simulink model "BldcClosedLoop2"  (R2020b)
settings: Solver=ode45  StartTime=0.0  StopTime=1  FixedStep=.001  RelTol=1e-3  AbsTol=1e-3  EnableMultiTasking=on
values from neighbouring files (symbols this model uses):
  c1 = 3*wmax/(t1*t1)    (= 120000)    [data_bldc_ClosedLoop2.m]
  c2 = -2*wmax/(t1*t1*t1)    (= -800000)    [data_bldc_ClosedLoop2.m]
  D = 2e-3    (= 0.002)    [data_bldc_ClosedLoop2.m]
  d1 = 3*wmax/((t3-t2)*(t3-t2))    (= 120000)    [data_bldc_ClosedLoop2.m]
  d2 = -2*wmax/((t3-t2)*(t3-t2)*(t3-t2))    (= -800000)    [data_bldc_ClosedLoop2.m]
  ep = 0.5128    [data_bldc_ClosedLoop2.m]
  Gamma_Inv = Gamma^-1    [data_bldc_ClosedLoop2.m]
  J = 2.0e-4    (= 0.0002)    [data_bldc_ClosedLoop2.m]
  k0 = p0*p1*p2    (= 1000000)    [data_bldc_ClosedLoop2.m]
  k1 = p0*p1 + p0*p2 + p1*p2    (= 30000)    [data_bldc_ClosedLoop2.m]
  k2 = p0+p1+p2    (= 300)    [data_bldc_ClosedLoop2.m]
  KI = 0*1e6    (= 0)    [data_bldc_ClosedLoop2.m]
  Kp = 1000    [data_bldc_ClosedLoop2.m]
  Rs = 0.7    [data_bldc_ClosedLoop2.m]
  t3 = t2 + t1    (= 0.7)    [data_bldc_ClosedLoop2.m]
  tau_L = 0    [data_bldc_ClosedLoop2.m]
  tdd = .1    (= 0.1)    [data_bldc_ClosedLoop2.m]
libraries: simulink x2
(part 1 of 2)
settings Model: Creator=johnchiasson  LastModifiedBy=johnchiasson
settings SolverCC: AutoScaleAbsTol=off
settings DataIOCC: LimitDataPoints=on  SaveFormat=Array  SignalLoggingSaveFormat=ModelDataLogs  ReturnWorkspaceOutputs=off  SignalLoggingName=sigsOut
settings OptimizationCC: BlockReduction=off  BooleanDataType=off  LifeSpan=inf
settings DebuggingCC: SaveWithParameterizedLinksMsg=none  UnderspecifiedInitializationDetection=Classic  MergeDetectMultiDrivingBlocksExec=none  SignalResolutionControl=TryResolveAllWithWarning  MultiTaskDSMMsg=warning  MultiTaskCondExecSysMsg=none  SFUnexpectedBacktrackingDiag=warning  SFNoUnconditionalDefaultTransitionDiag=warning  SFExecutionAtInitializationDiag=none  ArithmeticOperatorsInVariantConditions=warning
settings HardwareCC: ProdBitPerPointer=32  ProdBitPerSizeT=32  ProdBitPerPtrDiffT=32  ProdLargestAtomicFloat=None  ProdIntDivRoundTo=Undefined  ProdEndianess=Unspecified  ProdWordSize=32  ProdHWDeviceType=32-bit Generic  TargetUnknown=on
settings ModelReferenceCC: PropagateSignalLabelsOutOfModel=off
settings SFSimCC: SimUseLocalCustomCode=off  CustomCodeUndefinedFunction=UseInterfaceOnly
settings RTWCC: RTWUseLocalCustomCode=off
settings CodeAppCC: StateflowObjectComments=on
settings GRTTargetCC: TargetLangStandard=C89/C90 (ANSI)  CombineOutputUpdateFcns=off  GRTInterface=on
settings ConfigComp: CovMetricSettings=dw  CovSaveCumulativeToWorkspaceVar=on  CovSaveSingleToWorkspaceVar=on  CovExternalEMLEnable=off  CovSFcnEnable=off

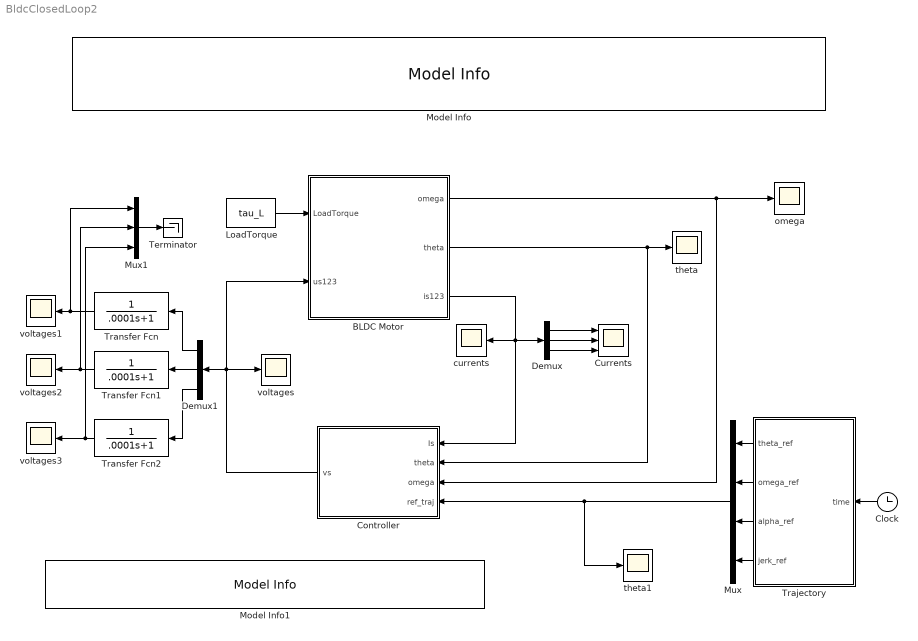
== system BldcClosedLoop2 ==
  BLDC Motor : Subsystem
  Clock : Clock
  Controller : Subsystem
  Currents : Scope  NumInputPorts=3
  Demux : Demux  Outputs=3
      settings: DisplayOption=none
  Demux1 : Demux  Outputs=3
      settings: DisplayOption=none
  LoadTorque : Constant  Value=tau_L
  Model Info : simulink/Model-Wide Utilities/Model Info  Frame=on  DisplayStringWithTags="Simulation of a Three-Phase  Trapezoidal Back EMF BLDC"  HorizontalTextAlignment=Center  LeftAlignmentValue=0.5
  Model Info1 : simulink/Model-Wide Utilities/Model Info  Frame=on  DisplayStringWithTags=|  HorizontalTextAlignment=Left  LeftAlignmentValue=0.02
      | Changed the gain in the torque from 1/ep to 1/(2ep) 
      | Replaced ep by -ep
  Mux : Mux
  Mux1 : Mux  Inputs=3
  Terminator : Terminator
  Trajectory : Subsystem
  Transfer Fcn : TransferFcn  Denominator=[.0001 1]
  Transfer Fcn1 : TransferFcn  Denominator=[.0001 1]
  Transfer Fcn2 : TransferFcn  Denominator=[.0001 1]
  currents : Scope
  omega : Scope
  theta : Scope
  theta1 : Scope
  voltages{,1..3} (4 alike) : Scope
  wires:
  BLDC Motor/3(is123) -> Controller/1(Is), currents/1, Demux/1
  BLDC Motor/1(omega) -> Controller/3(omega), omega/1
  Controller/1(vs) -> voltages/1, Demux1/1, BLDC Motor/2(us123)
  Clock/1 -> Trajectory/1(time)
  Mux/1 -> theta1/1, Controller/4(ref_traj)
  Trajectory/4(jerk_ref) -> Mux/4
  Trajectory/1(theta_ref) -> Mux/1
  Trajectory/2(omega_ref) -> Mux/2
  Trajectory/3(alpha_ref) -> Mux/3
  BLDC Motor/2(theta) -> Controller/2(theta), theta/1
  Demux/1 -> Currents/1
  Demux1/1 -> Transfer Fcn/1
  Transfer Fcn/1 -> voltages1/1, Mux1/1
  Demux/2 -> Currents/2
  Demux/3 -> Currents/3
  Transfer Fcn1/1 -> voltages2/1, Mux1/2
  Demux1/2 -> Transfer Fcn1/1
  Transfer Fcn2/1 -> voltages3/1, Mux1/3
  Demux1/3 -> Transfer Fcn2/1
  LoadTorque/1 -> BLDC Motor/1(LoadTorque)
  Mux1/1 -> Terminator/1

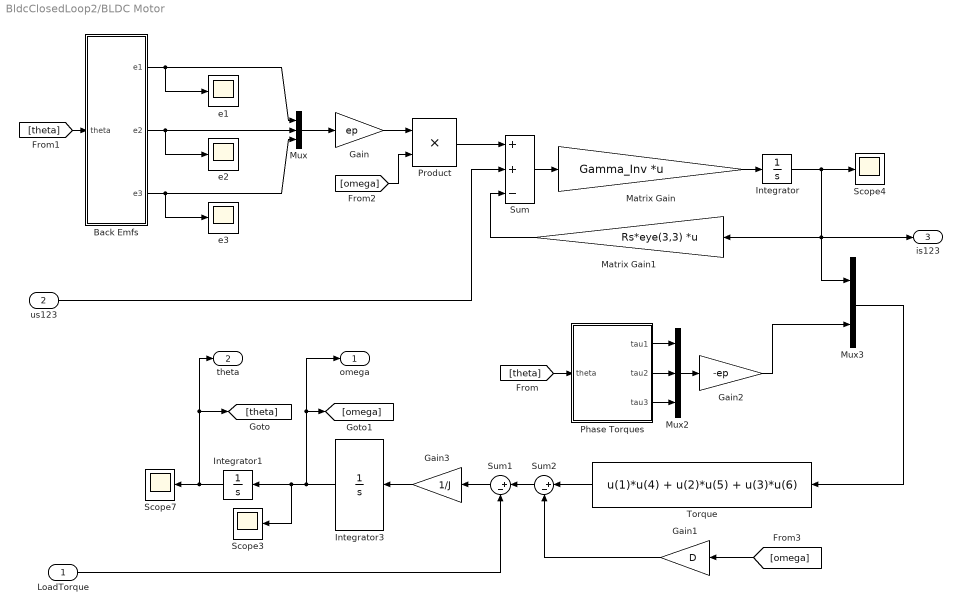
== system BldcClosedLoop2/BLDC Motor ==
  LoadTorque : Inport
  us123 : Inport  Port=2
  Back Emfs : Subsystem
  Gain : Gain  Gain=ep  SaturateOnIntegerOverflow=on  OutDataTypeStr=Inherit: Same as input  ParamDataTypeStr=Inherit: Same as input
  Gain1 : Gain  Gain=D  SaturateOnIntegerOverflow=on  OutDataTypeStr=Inherit: Same as input  ParamDataTypeStr=Inherit: Same as input
  Gain2 : Gain  Gain=-ep  SaturateOnIntegerOverflow=on  OutDataTypeStr=Inherit: Same as input  ParamDataTypeStr=Inherit: Same as input
  Gain3 : Gain  Gain=1/J  SaturateOnIntegerOverflow=on  OutDataTypeStr=Inherit: Same as input  ParamDataTypeStr=Inherit: Same as input
  Integrator : Integrator
  Integrator1 : Integrator
  Integrator3 : Integrator
  Matrix Gain : Gain  Gain=Gamma_Inv  Multiplication=Matrix(K*u)  SaturateOnIntegerOverflow=on  OutDataTypeStr=Inherit: Same as input  ParamDataTypeStr=Inherit: Same as input
  Matrix Gain1 : Gain  Gain=Rs*eye(3,3)  Multiplication=Matrix(K*u)  SaturateOnIntegerOverflow=on  OutDataTypeStr=Inherit: Same as input  ParamDataTypeStr=Inherit: Same as input
  Mux : Mux  Inputs=3
  Mux2 : Mux  Inputs=3
  Mux3 : Mux  Inputs=2
  Phase Torques : Subsystem
  Product : Product  InputSameDT=on  SaturateOnIntegerOverflow=on  OutDataTypeStr=Inherit: Same as first input
  Scope3 : Scope
  Scope4 : Scope
  Scope7 : Scope
  Sum : Sum  Inputs=++-  InputSameDT=on  SaturateOnIntegerOverflow=on  OutDataTypeStr=Inherit: Same as first input
  Sum1 : Sum  Inputs=|+-  InputSameDT=on  SaturateOnIntegerOverflow=on  OutDataTypeStr=Inherit: Same as first input
  Sum2 : Sum  Inputs=|+-  InputSameDT=on  SaturateOnIntegerOverflow=on  OutDataTypeStr=Inherit: Same as first input
  Torque : Fcn  Expr=u(1)*u(4) + u(2)*u(5) + u(3)*u(6)
  e1 : Scope
  e2 : Scope
  e3 : Scope
  omega : Outport
  theta : Outport  Port=2
  is123 : Outport  Port=3
  wires:
  Back Emfs/1(e1) -> e1/1, Mux/1
  Back Emfs/2(e2) -> e2/1, Mux/2
  Back Emfs/3(e3) -> e3/1, Mux/3
  Mux/1 -> Gain/1
  Gain/1 -> Product/1
  Integrator/1 -> Scope4/1, Mux3/1, is123/1, Matrix Gain1/1
  [omega] -> Product/2
  Matrix Gain/1 -> Integrator/1
  Product/1 -> Sum/1
  Sum/1 -> Matrix Gain/1
  Matrix Gain1/1 -> Sum/3
  Phase Torques/2(tau2) -> Mux2/2
  Phase Torques/1(tau1) -> Mux2/1
  Phase Torques/3(tau3) -> Mux2/3
  Mux2/1 -> Gain2/1
  Gain2/1 -> Mux3/2
  Mux3/1 -> Torque/1
  Gain3/1 -> Integrator3/1
  Integrator1/1 -> Scope7/1, [theta], theta/1
  [theta] -> Phase Torques/1(theta)
  [theta] -> Back Emfs/1(theta)
  Integrator3/1 -> Scope3/1, Integrator1/1, [omega], omega/1
  us123/1 -> Sum/2
  [omega] -> Gain1/1
  Torque/1 -> Sum2/1
  Gain1/1 -> Sum2/2
  Sum1/1 -> Gain3/1
  Sum2/1 -> Sum1/1
  LoadTorque/1 -> Sum1/2

== system BldcClosedLoop2/Controller ==
  Is : Inport
  theta : Inport  Port=2
  omega : Inport  Port=3
  ref_traj : Inport  Port=4
  Current Controller : Subsystem
  Demux : Demux  Outputs=3
      settings: DisplayOption=none
  Gain1 : Gain  Gain=1/(2*ep)  SaturateOnIntegerOverflow=on  OutDataTypeStr=Inherit: Same as input  ParamDataTypeStr=Inherit: Same as input
  Product : Product  InputSameDT=on  SaturateOnIntegerOverflow=on  OutDataTypeStr=Inherit: Same as first input
  Traj_Tracking_Controller : Subsystem
  current commands : Subsystem
  isc1 : Scope
  isc2 : Scope
  isc3 : Scope
  vs : Outport
  wires:
  Product/1 -> Current Controller/2(isc), Demux/1
  Gain1/1 -> Product/2
  current commands/1(isc) -> Product/1
  Traj_Tracking_Controller/1(Torque_Command) -> Gain1/1
  theta/1 -> current commands/1(theta), Traj_Tracking_Controller/1(theta)
  Is/1 -> Current Controller/1(is)
  Current Controller/1(vs123) -> vs/1
  omega/1 -> Traj_Tracking_Controller/2(omega)
  ref_traj/1 -> Traj_Tracking_Controller/3(ref_traj)
  Demux/1 -> isc1/1
  Demux/2 -> isc2/1
  Demux/3 -> isc3/1

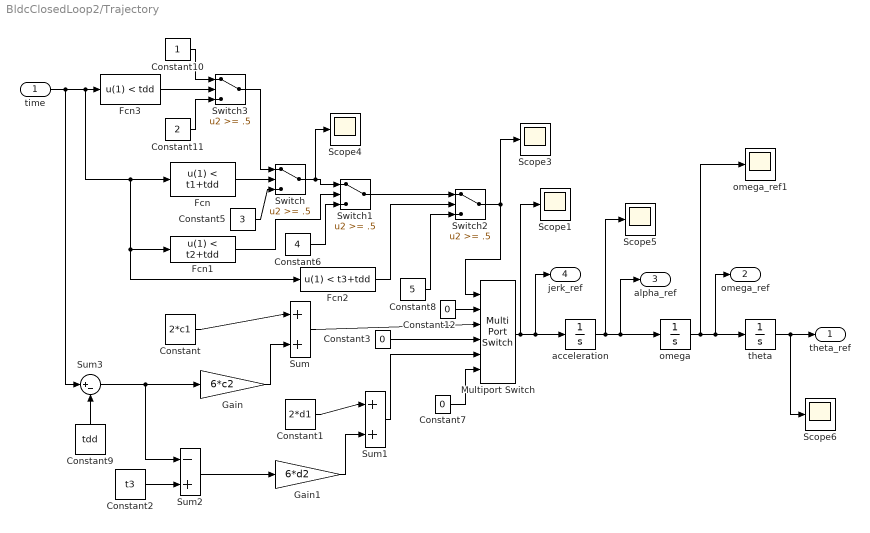
== system BldcClosedLoop2/Trajectory ==
  time : Inport
  Constant : Constant  Value=2*c1
  Constant1 : Constant  Value=2*d1
  Constant10 : Constant
  Constant11 : Constant  Value=2
  Constant12 : Constant  Value=0
  Constant2 : Constant  Value=t3
  Constant3 : Constant  Value=0
  Constant5 : Constant  Value=3
  Constant6 : Constant  Value=4
  Constant7 : Constant  Value=0
  Constant8 : Constant  Value=5
  Constant9 : Constant  Value=tdd
  Fcn : Fcn  Expr=u(1) < t1+tdd
  Fcn1 : Fcn  Expr=u(1) < t2+tdd
  Fcn2 : Fcn  Expr=u(1) < t3+tdd
  Fcn3 : Fcn  Expr=u(1) < tdd
  Gain : Gain  Gain=6*c2  SaturateOnIntegerOverflow=on  OutDataTypeStr=Inherit: Same as input  ParamDataTypeStr=Inherit: Same as input
  Gain1 : Gain  Gain=6*d2  SaturateOnIntegerOverflow=on  OutDataTypeStr=Inherit: Same as input  ParamDataTypeStr=Inherit: Same as input
  Multiport Switch : MultiPortSwitch  Inputs=5  SaturateOnIntegerOverflow=on  InputSameDT=on
  Scope{1,3..6} (5 alike) : Scope
  Sum : Sum  Inputs=|++  InputSameDT=on  SaturateOnIntegerOverflow=on  OutDataTypeStr=Inherit: Same as first input
  Sum1 : Sum  Inputs=|++  InputSameDT=on  SaturateOnIntegerOverflow=on  OutDataTypeStr=Inherit: Same as first input
  Sum2 : Sum  Inputs=-+  InputSameDT=on  SaturateOnIntegerOverflow=on  OutDataTypeStr=Inherit: Same as first input
  Sum3 : Sum  Inputs=|+-  InputSameDT=on  SaturateOnIntegerOverflow=on  OutDataTypeStr=Inherit: Same as first input
  Switch{,1..3} (4 alike) : Switch  Threshold=.5  SaturateOnIntegerOverflow=on  InputSameDT=on
  acceleration : Integrator
  omega : Integrator
  omega_ref1 : Scope
  theta : Integrator
  theta_ref : Outport
  omega_ref : Outport  Port=2
  alpha_ref : Outport  Port=3
  jerk_ref : Outport  Port=4
  wires:
  Constant/1 -> Sum/1
  Gain/1 -> Sum/2
  Constant2/1 -> Sum2/2
  Sum2/1 -> Gain1/1
  Constant1/1 -> Sum1/1
  Gain1/1 -> Sum1/2
  Fcn/1 -> Switch/2
  Constant5/1 -> Switch/3
  Constant6/1 -> Switch1/3
  Fcn1/1 -> Switch1/2
  Switch/1 -> Switch1/1, Scope4/1
  Sum1/1 -> Multiport Switch/5
  Sum/1 -> Multiport Switch/3
  Constant3/1 -> Multiport Switch/4
  omega/1 -> theta/1, omega_ref/1, omega_ref1/1
  Multiport Switch/1 -> acceleration/1, jerk_ref/1, Scope1/1
  acceleration/1 -> omega/1, alpha_ref/1, Scope5/1
  theta/1 -> theta_ref/1, Scope6/1
  Constant7/1 -> Multiport Switch/6
  Fcn2/1 -> Switch2/2
  Constant8/1 -> Switch2/3
  Switch1/1 -> Switch2/1
  Switch2/1 -> Scope3/1, Multiport Switch/1
  Constant12/1 -> Multiport Switch/2
  Switch3/1 -> Switch/1
  Constant10/1 -> Switch3/1
  Constant11/1 -> Switch3/3
  Fcn3/1 -> Switch3/2
  Constant9/1 -> Sum3/2
  Sum3/1 -> Gain/1, Sum2/1
  time/1 -> Fcn3/1, Fcn/1, Fcn1/1, Fcn2/1, Sum3/1

== system BldcClosedLoop2/BLDC Motor/Back Emfs ==
  theta : Inport
  Constant1 : Constant  Value=2*pi/3
  Constant2 : Constant  Value=4*pi/3
  Sum : Sum  Inputs=|+-  InputSameDT=on  SaturateOnIntegerOverflow=on  OutDataTypeStr=Inherit: Same as first input
  Sum1 : Sum  Inputs=|+-  InputSameDT=on  SaturateOnIntegerOverflow=on  OutDataTypeStr=Inherit: Same as first input
  es1 : Subsystem
  es2 : Subsystem
  es3 : Subsystem
  e1 : Outport
  e2 : Outport  Port=2
  e3 : Outport  Port=3
  wires:
  Constant1/1 -> Sum/2
  Sum/1 -> es2/1(theta)
  Constant2/1 -> Sum1/2
  Sum1/1 -> es3/1(theta)
  es1/1(e1) -> e1/1
  theta/1 -> es1/1(theta), Sum/1, Sum1/1
  es2/1(e2) -> e2/1
  es3/1(e3) -> e3/1

== system BldcClosedLoop2/BLDC Motor/Phase Torques ==
  theta : Inport
  Constant1 : Constant  Value=2*pi/3
  Constant2 : Constant  Value=4*pi/3
  Sum : Sum  Inputs=|+-  InputSameDT=on  SaturateOnIntegerOverflow=on  OutDataTypeStr=Inherit: Same as first input
  Sum1 : Sum  Inputs=|+-  InputSameDT=on  SaturateOnIntegerOverflow=on  OutDataTypeStr=Inherit: Same as first input
  Tau1 : Subsystem
  Tau2 : Subsystem
  Tau3 : Subsystem
  tau1 : Outport
  tau2 : Outport  Port=2
  tau3 : Outport  Port=3
  wires:
  Constant1/1 -> Sum/2
  Sum/1 -> Tau2/1(theta)
  Constant2/1 -> Sum1/2
  Sum1/1 -> Tau3/1(theta)
  Tau1/1(tau1) -> tau1/1
  theta/1 -> Tau1/1(theta), Sum/1, Sum1/1
  Tau2/1(tau2) -> tau2/1
  Tau3/1(tau3) -> tau3/1

== system BldcClosedLoop2/Controller/Current Controller ==
  is : Inport
  isc : Inport  Port=2
  Gain13 : Gain  Gain=KI  SaturateOnIntegerOverflow=on  OutDataTypeStr=Inherit: Same as input  ParamDataTypeStr=Inherit: Same as input
  Gain14 : Gain  Gain=Kp  SaturateOnIntegerOverflow=on  OutDataTypeStr=Inherit: Same as input  ParamDataTypeStr=Inherit: Same as input
  Integrator4 : Integrator
  Scope5 : Scope
  Sum4 : Sum  Inputs=-+  InputSameDT=on  SaturateOnIntegerOverflow=on  OutDataTypeStr=Inherit: Same as first input
  Sum6 : Sum  InputSameDT=on  SaturateOnIntegerOverflow=on  OutDataTypeStr=Inherit: Same as first input
  vs123 : Outport
  wires:
  Sum4/1 -> Scope5/1, Gain14/1, Gain13/1
  Gain13/1 -> Integrator4/1
  is/1 -> Sum4/1
  isc/1 -> Sum4/2
  Integrator4/1 -> Sum6/2
  Gain14/1 -> Sum6/1
  Sum6/1 -> vs123/1

== system BldcClosedLoop2/Controller/Traj_Tracking_Controller ==
  theta : Inport
  omega : Inport  Port=2
  ref_traj : Inport  Port=3
  Demux : Demux
      settings: DisplayOption=none
  Gain2 : Gain  Gain=k0  SaturateOnIntegerOverflow=on  OutDataTypeStr=Inherit: Same as input  ParamDataTypeStr=Inherit: Same as input
  Gain3 : Gain  Gain=k1  SaturateOnIntegerOverflow=on  OutDataTypeStr=Inherit: Same as input  ParamDataTypeStr=Inherit: Same as input
  Gain4 : Gain  Gain=k2  SaturateOnIntegerOverflow=on  OutDataTypeStr=Inherit: Same as input  ParamDataTypeStr=Inherit: Same as input
  Gain5 : Gain  Gain=J  SaturateOnIntegerOverflow=on  OutDataTypeStr=Inherit: Same as input  ParamDataTypeStr=Inherit: Same as input
  Integrator : Integrator
  Scope3 : Scope
  Scope4 : Scope
  Scope5 : Scope
  Sum1 : Sum  Inputs=+-  InputSameDT=on  SaturateOnIntegerOverflow=on  OutDataTypeStr=Inherit: Same as first input
  Sum2 : Sum  Inputs=+-  InputSameDT=on  SaturateOnIntegerOverflow=on  OutDataTypeStr=Inherit: Same as first input
  Sum3 : Sum  Inputs=++++  InputSameDT=on  SaturateOnIntegerOverflow=on  OutDataTypeStr=Inherit: Same as first input
  Terminator : Terminator
  Torque_Command : Outport
  wires:
  Demux/1 -> Sum1/1
  Gain2/1 -> Integrator/1
  Integrator/1 -> Sum3/1
  theta/1 -> Sum1/2
  ref_traj/1 -> Demux/1
  Demux/4 -> Terminator/1
  Demux/2 -> Sum2/1
  Gain4/1 -> Sum3/3
  Sum3/1 -> Gain5/1
  Sum1/1 -> Gain2/1, Gain3/1, Scope3/1
  Sum2/1 -> Gain4/1, Scope4/1
  Gain3/1 -> Sum3/2, Scope5/1
  Gain5/1 -> Torque_Command/1
  omega/1 -> Sum2/2
  Demux/3 -> Sum3/4

== system BldcClosedLoop2/Controller/current commands ==
  theta : Inport
  Constant1 : Constant  Value=2*pi/3
  Constant2 : Constant  Value=4*pi/3
  IS1c : Subsystem
  IS2c : Subsystem
  IS3c : Subsystem
  Mux3 : Mux  Inputs=3
  Sum : Sum  Inputs=|+-  InputSameDT=on  SaturateOnIntegerOverflow=on  OutDataTypeStr=Inherit: Same as first input
  Sum1 : Sum  Inputs=|+-  InputSameDT=on  SaturateOnIntegerOverflow=on  OutDataTypeStr=Inherit: Same as first input
  isc : Outport
  wires:
  Constant1/1 -> Sum/2
  Sum/1 -> IS2c/1(theta)
  Constant2/1 -> Sum1/2
  Sum1/1 -> IS3c/1(theta)
  IS1c/1(is1c) -> Mux3/1
  theta/1 -> IS1c/1(theta), Sum/1, Sum1/1
  IS2c/1(is2c) -> Mux3/2
  IS3c/1(is3c) -> Mux3/3
  Mux3/1 -> isc/1

== system BldcClosedLoop2/BLDC Motor/Back Emfs/es1 ==
  theta : Inport
  "-pi/6 < theta < 11pi/6 " : Subsystem
  0 < theta < 2pi : Subsystem
  Constant : Constant
  Constant1 : Constant  Value=-1
  Constant2 : Constant  Value=pi
  Gain1 : Gain  Gain=6/pi  SaturateOnIntegerOverflow=on  OutDataTypeStr=Inherit: Same as input  ParamDataTypeStr=Inherit: Same as input
  Gain2 : Gain  Gain=-6/pi  SaturateOnIntegerOverflow=on  OutDataTypeStr=Inherit: Same as input  ParamDataTypeStr=Inherit: Same as input
  Multiport Switch : MultiPortSwitch  Inputs=4  SaturateOnIntegerOverflow=on  InputSameDT=on
  Sum2 : Sum  Inputs=|+-  InputSameDT=on  SaturateOnIntegerOverflow=on  OutDataTypeStr=Inherit: Same as first input
  interval : Subsystem
  e1 : Outport
  wires:
  interval/1(interval) -> Multiport Switch/1
  Multiport Switch/1 -> e1/1
  Gain1/1 -> Multiport Switch/2
  Constant/1 -> Multiport Switch/3
  Constant1/1 -> Multiport Switch/5
  Constant2/1 -> Sum2/2
  0 < theta < 2pi/1(0 < theta < 2pi) -> "-pi/6 < theta < 11pi/6 "/1(0 < theta < 2pi)
  Gain2/1 -> Multiport Switch/4
  Sum2/1 -> Gain2/1
  theta/1 -> 0 < theta < 2pi/1(theta)
  "-pi/6 < theta < 11pi/6 "/1(-pi/6 < theta < 11pi/6) -> Gain1/1, Sum2/1, interval/1(-pi/6 < theta < 11pi/6)

== system BldcClosedLoop2/BLDC Motor/Back Emfs/es2 ==
  theta : Inport
  -pi/6 < theta < 11pi/6 : Subsystem
  0 < theta < 2pi : Subsystem
  Constant : Constant
  Constant1 : Constant  Value=-1
  Constant2 : Constant  Value=pi
  Gain1 : Gain  Gain=6/pi  SaturateOnIntegerOverflow=on  OutDataTypeStr=Inherit: Same as input  ParamDataTypeStr=Inherit: Same as input
  Gain2 : Gain  Gain=-6/pi  SaturateOnIntegerOverflow=on  OutDataTypeStr=Inherit: Same as input  ParamDataTypeStr=Inherit: Same as input
  Multiport Switch : MultiPortSwitch  Inputs=4  SaturateOnIntegerOverflow=on  InputSameDT=on
  Sum2 : Sum  Inputs=|+-  InputSameDT=on  SaturateOnIntegerOverflow=on  OutDataTypeStr=Inherit: Same as first input
  interval : Subsystem
  e2 : Outport
  wires:
  interval/1(interval) -> Multiport Switch/1
  Multiport Switch/1 -> e2/1
  Gain1/1 -> Multiport Switch/2
  Constant/1 -> Multiport Switch/3
  Constant1/1 -> Multiport Switch/5
  Constant2/1 -> Sum2/2
  0 < theta < 2pi/1(0 < theta < 2pi) -> -pi/6 < theta < 11pi/6/1(0 < theta < 2pi)
  Gain2/1 -> Multiport Switch/4
  Sum2/1 -> Gain2/1
  theta/1 -> 0 < theta < 2pi/1(theta)
  -pi/6 < theta < 11pi/6/1(-pi/6 < theta < 11pi/6) -> Gain1/1, Sum2/1, interval/1(-pi/6 < theta < 11pi/6)

== system BldcClosedLoop2/BLDC Motor/Back Emfs/es3 ==
  theta : Inport
  -pi/6 < theta < 11pi/6 : Subsystem
  0 < theta < 2pi : Subsystem
  Constant : Constant
  Constant1 : Constant  Value=-1
  Constant2 : Constant  Value=pi
  Gain1 : Gain  Gain=6/pi  SaturateOnIntegerOverflow=on  OutDataTypeStr=Inherit: Same as input  ParamDataTypeStr=Inherit: Same as input
  Gain2 : Gain  Gain=-6/pi  SaturateOnIntegerOverflow=on  OutDataTypeStr=Inherit: Same as input  ParamDataTypeStr=Inherit: Same as input
  Multiport Switch : MultiPortSwitch  Inputs=4  SaturateOnIntegerOverflow=on  InputSameDT=on
  Sum2 : Sum  Inputs=|+-  InputSameDT=on  SaturateOnIntegerOverflow=on  OutDataTypeStr=Inherit: Same as first input
  interval : Subsystem
  e3 : Outport
  wires:
  interval/1(interval) -> Multiport Switch/1
  Multiport Switch/1 -> e3/1
  Gain1/1 -> Multiport Switch/2
  Constant/1 -> Multiport Switch/3
  Constant1/1 -> Multiport Switch/5
  Constant2/1 -> Sum2/2
  0 < theta < 2pi/1(0 < theta < 2pi) -> -pi/6 < theta < 11pi/6/1(0 < theta < 2pi)
  Gain2/1 -> Multiport Switch/4
  Sum2/1 -> Gain2/1
  theta/1 -> 0 < theta < 2pi/1(theta)
  -pi/6 < theta < 11pi/6/1(-pi/6 < theta < 11pi/6) -> Gain1/1, Sum2/1, interval/1(-pi/6 < theta < 11pi/6)

== system BldcClosedLoop2/BLDC Motor/Phase Torques/Tau1 ==
  theta : Inport
  "-pi/6 < theta < 11pi/6 " : Subsystem
  0 < theta < 2pi : Subsystem
  Constant : Constant
  Constant1 : Constant  Value=-1
  Constant2 : Constant  Value=pi
  Gain1 : Gain  Gain=6/pi  SaturateOnIntegerOverflow=on  OutDataTypeStr=Inherit: Same as input  ParamDataTypeStr=Inherit: Same as input
  Gain2 : Gain  Gain=-6/pi  SaturateOnIntegerOverflow=on  OutDataTypeStr=Inherit: Same as input  ParamDataTypeStr=Inherit: Same as input
  Multiport Switch : MultiPortSwitch  Inputs=4  SaturateOnIntegerOverflow=on  InputSameDT=on
  Sum2 : Sum  Inputs=|+-  InputSameDT=on  SaturateOnIntegerOverflow=on  OutDataTypeStr=Inherit: Same as first input
  interval : Subsystem
  tau1 : Outport
  wires:
  interval/1(interval) -> Multiport Switch/1
  Multiport Switch/1 -> tau1/1
  Gain1/1 -> Multiport Switch/2
  Constant/1 -> Multiport Switch/3
  Constant1/1 -> Multiport Switch/5
  Constant2/1 -> Sum2/2
  0 < theta < 2pi/1(0 < theta < 2pi) -> "-pi/6 < theta < 11pi/6 "/1(0 < theta < 2pi)
  Gain2/1 -> Multiport Switch/4
  Sum2/1 -> Gain2/1
  theta/1 -> 0 < theta < 2pi/1(theta)
  "-pi/6 < theta < 11pi/6 "/1(-pi/6 < theta < 11pi/6) -> Gain1/1, Sum2/1, interval/1(-pi/6 < theta < 11pi/6)

== system BldcClosedLoop2/BLDC Motor/Phase Torques/Tau2 ==
  theta : Inport
  -pi/6 < theta < 11pi/6 : Subsystem
  0 < theta < 2pi : Subsystem
  Constant : Constant
  Constant1 : Constant  Value=-1
  Constant2 : Constant  Value=pi
  Gain1 : Gain  Gain=6/pi  SaturateOnIntegerOverflow=on  OutDataTypeStr=Inherit: Same as input  ParamDataTypeStr=Inherit: Same as input
  Gain2 : Gain  Gain=-6/pi  SaturateOnIntegerOverflow=on  OutDataTypeStr=Inherit: Same as input  ParamDataTypeStr=Inherit: Same as input
  Multiport Switch : MultiPortSwitch  Inputs=4  SaturateOnIntegerOverflow=on  InputSameDT=on
  Sum2 : Sum  Inputs=|+-  InputSameDT=on  SaturateOnIntegerOverflow=on  OutDataTypeStr=Inherit: Same as first input
  interval : Subsystem
  tau2 : Outport
  wires:
  interval/1(interval) -> Multiport Switch/1
  Multiport Switch/1 -> tau2/1
  Gain1/1 -> Multiport Switch/2
  Constant/1 -> Multiport Switch/3
  Constant1/1 -> Multiport Switch/5
  Constant2/1 -> Sum2/2
  0 < theta < 2pi/1(0 < theta < 2pi) -> -pi/6 < theta < 11pi/6/1(0 < theta < 2pi)
  Gain2/1 -> Multiport Switch/4
  Sum2/1 -> Gain2/1
  theta/1 -> 0 < theta < 2pi/1(theta)
  -pi/6 < theta < 11pi/6/1(-pi/6 < theta < 11pi/6) -> Gain1/1, Sum2/1, interval/1(-pi/6 < theta < 11pi/6)

== system BldcClosedLoop2/BLDC Motor/Phase Torques/Tau3 ==
  theta : Inport
  -pi/6 < theta < 11pi/6 : Subsystem
  0 < theta < 2pi : Subsystem
  Constant : Constant
  Constant1 : Constant  Value=-1
  Constant2 : Constant  Value=pi
  Gain1 : Gain  Gain=6/pi  SaturateOnIntegerOverflow=on  OutDataTypeStr=Inherit: Same as input  ParamDataTypeStr=Inherit: Same as input
  Gain2 : Gain  Gain=-6/pi  SaturateOnIntegerOverflow=on  OutDataTypeStr=Inherit: Same as input  ParamDataTypeStr=Inherit: Same as input
  Multiport Switch : MultiPortSwitch  Inputs=4  SaturateOnIntegerOverflow=on  InputSameDT=on
  Sum2 : Sum  Inputs=|+-  InputSameDT=on  SaturateOnIntegerOverflow=on  OutDataTypeStr=Inherit: Same as first input
  interval : Subsystem
  tau3 : Outport
  wires:
  interval/1(interval) -> Multiport Switch/1
  Multiport Switch/1 -> tau3/1
  Gain1/1 -> Multiport Switch/2
  Constant/1 -> Multiport Switch/3
  Constant1/1 -> Multiport Switch/5
  Constant2/1 -> Sum2/2
  0 < theta < 2pi/1(0 < theta < 2pi) -> -pi/6 < theta < 11pi/6/1(0 < theta < 2pi)
  Gain2/1 -> Multiport Switch/4
  Sum2/1 -> Gain2/1
  theta/1 -> 0 < theta < 2pi/1(theta)
  -pi/6 < theta < 11pi/6/1(-pi/6 < theta < 11pi/6) -> Gain1/1, Sum2/1, interval/1(-pi/6 < theta < 11pi/6)

== system BldcClosedLoop2/Controller/current commands/IS1c ==
  theta : Inport
  "-pi/6 < theta < 11pi/6 " : Subsystem
  0 < theta < 2pi : Subsystem
  Constant : Constant  Value=-1
  Constant1 : Constant
  Constant2 : Constant  Value=pi
  Gain1 : Gain  Gain=0  SaturateOnIntegerOverflow=on  OutDataTypeStr=Inherit: Same as input  ParamDataTypeStr=Inherit: Same as input
  Gain2 : Gain  Gain=0  SaturateOnIntegerOverflow=on  OutDataTypeStr=Inherit: Same as input  ParamDataTypeStr=Inherit: Same as input
  Multiport Switch : MultiPortSwitch  Inputs=4  SaturateOnIntegerOverflow=on  InputSameDT=on
  Sum2 : Sum  Inputs=|+-  InputSameDT=on  SaturateOnIntegerOverflow=on  OutDataTypeStr=Inherit: Same as first input
  interval : Subsystem
  is1c : Outport
  wires:
  interval/1(interval) -> Multiport Switch/1
  Multiport Switch/1 -> is1c/1
  Gain1/1 -> Multiport Switch/2
  Constant/1 -> Multiport Switch/3
  Constant1/1 -> Multiport Switch/5
  Constant2/1 -> Sum2/2
  0 < theta < 2pi/1(0 < theta < 2pi) -> "-pi/6 < theta < 11pi/6 "/1(0 < theta < 2pi)
  Gain2/1 -> Multiport Switch/4
  Sum2/1 -> Gain2/1
  theta/1 -> 0 < theta < 2pi/1(theta)
  "-pi/6 < theta < 11pi/6 "/1(-pi/6 < theta < 11pi/6) -> Gain1/1, Sum2/1, interval/1(-pi/6 < theta < 11pi/6)

== system BldcClosedLoop2/Controller/current commands/IS2c ==
  theta : Inport
  -pi/6 < theta < 11pi/6 : Subsystem
  0 < theta < 2pi : Subsystem
  Constant : Constant  Value=-1
  Constant1 : Constant
  Constant2 : Constant  Value=pi
  Gain1 : Gain  Gain=0  SaturateOnIntegerOverflow=on  OutDataTypeStr=Inherit: Same as input  ParamDataTypeStr=Inherit: Same as input
  Gain2 : Gain  Gain=0  SaturateOnIntegerOverflow=on  OutDataTypeStr=Inherit: Same as input  ParamDataTypeStr=Inherit: Same as input
  Multiport Switch : MultiPortSwitch  Inputs=4  SaturateOnIntegerOverflow=on  InputSameDT=on
  Sum2 : Sum  Inputs=|+-  InputSameDT=on  SaturateOnIntegerOverflow=on  OutDataTypeStr=Inherit: Same as first input
  interval : Subsystem
  is2c : Outport
  wires:
  interval/1(interval) -> Multiport Switch/1
  Multiport Switch/1 -> is2c/1
  Gain1/1 -> Multiport Switch/2
  Constant/1 -> Multiport Switch/3
  Constant1/1 -> Multiport Switch/5
  Constant2/1 -> Sum2/2
  0 < theta < 2pi/1(0 < theta < 2pi) -> -pi/6 < theta < 11pi/6/1(0 < theta < 2pi)
  Gain2/1 -> Multiport Switch/4
  Sum2/1 -> Gain2/1
  theta/1 -> 0 < theta < 2pi/1(theta)
  -pi/6 < theta < 11pi/6/1(-pi/6 < theta < 11pi/6) -> Gain1/1, Sum2/1, interval/1(-pi/6 < theta < 11pi/6)

== system BldcClosedLoop2/Controller/current commands/IS3c ==
  theta : Inport
  -pi/6 < theta < 11pi/6 : Subsystem
  0 < theta < 2pi : Subsystem
  Constant : Constant  Value=-1
  Constant1 : Constant
  Constant2 : Constant  Value=pi
  Gain1 : Gain  Gain=0  SaturateOnIntegerOverflow=on  OutDataTypeStr=Inherit: Same as input  ParamDataTypeStr=Inherit: Same as input
  Gain2 : Gain  Gain=0  SaturateOnIntegerOverflow=on  OutDataTypeStr=Inherit: Same as input  ParamDataTypeStr=Inherit: Same as input
  Multiport Switch : MultiPortSwitch  Inputs=4  SaturateOnIntegerOverflow=on  InputSameDT=on
  Sum2 : Sum  Inputs=|+-  InputSameDT=on  SaturateOnIntegerOverflow=on  OutDataTypeStr=Inherit: Same as first input
  interval : Subsystem
  is3c : Outport
  wires:
  interval/1(interval) -> Multiport Switch/1
  Multiport Switch/1 -> is3c/1
  Gain1/1 -> Multiport Switch/2
  Constant/1 -> Multiport Switch/3
  Constant1/1 -> Multiport Switch/5
  Constant2/1 -> Sum2/2
  0 < theta < 2pi/1(0 < theta < 2pi) -> -pi/6 < theta < 11pi/6/1(0 < theta < 2pi)
  Gain2/1 -> Multiport Switch/4
  Sum2/1 -> Gain2/1
  theta/1 -> 0 < theta < 2pi/1(theta)
  -pi/6 < theta < 11pi/6/1(-pi/6 < theta < 11pi/6) -> Gain1/1, Sum2/1, interval/1(-pi/6 < theta < 11pi/6)

== system BldcClosedLoop2/BLDC Motor/Back Emfs/es1/-pi//6 < theta < 11pi//6  ==
  0 < theta < 2pi : Inport
  Constant3 : Constant  Value=2*pi
  Fcn3 : Fcn  Expr="2*pi - u(1) <=  pi/6"
  Sum1 : Sum  Inputs=|-+  InputSameDT=on  SaturateOnIntegerOverflow=on  OutDataTypeStr=Inherit: Same as first input
  Switch1 : Switch  Threshold=.5  SaturateOnIntegerOverflow=on  InputSameDT=on
  -pi/6 < theta < 11pi/6 : Outport
  wires:
  0 < theta < 2pi/1 -> Switch1/3, Fcn3/1, Sum1/2
  Constant3/1 -> Sum1/1
  Switch1/1 -> -pi/6 < theta < 11pi/6/1
  Sum1/1 -> Switch1/1
  Fcn3/1 -> Switch1/2

== system BldcClosedLoop2/BLDC Motor/Back Emfs/es1/0 < theta < 2pi ==
  theta : Inport
  Constant1 : Constant  Value=2*pi
  Fcn4 : Fcn  Expr=rem(u(1),2*pi)
  Scope1 : Scope
  Sum2 : Sum  Inputs=|++  InputSameDT=on  SaturateOnIntegerOverflow=on  OutDataTypeStr=Inherit: Same as first input
  Switch3 : Switch  SaturateOnIntegerOverflow=on  InputSameDT=on
  0 < theta < 2pi : Outport
  wires:
  Sum2/1 -> Switch3/3
  Fcn4/1 -> Sum2/1, Switch3/1, Switch3/2
  Constant1/1 -> Sum2/2
  theta/1 -> Fcn4/1, Scope1/1
  Switch3/1 -> 0 < theta < 2pi/1

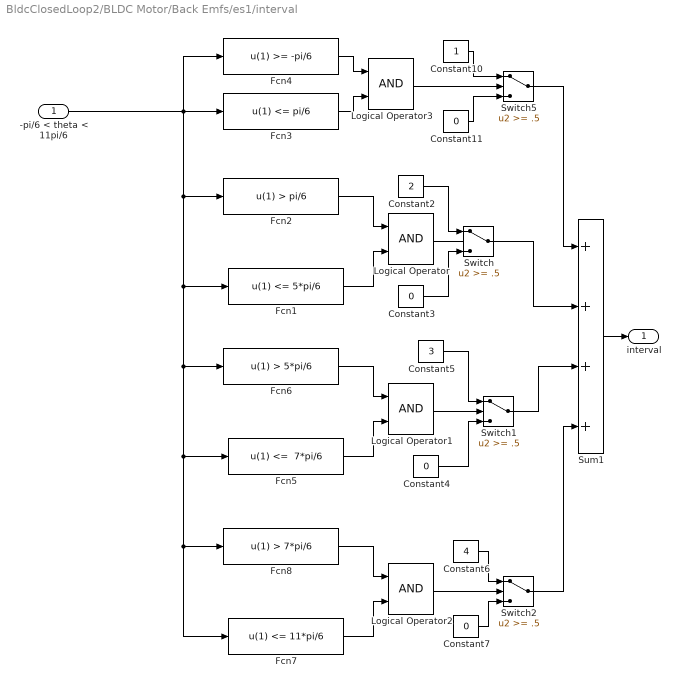
== system BldcClosedLoop2/BLDC Motor/Back Emfs/es1/interval ==
  -pi/6 < theta < 11pi/6 : Inport
  Constant10 : Constant
  Constant{3..4,7,11} (4 alike) : Constant  Value=0
  Constant2 : Constant  Value=2
  Constant5 : Constant  Value=3
  Constant6 : Constant  Value=4
  Fcn1 : Fcn  Expr=u(1) <= 5*pi/6
  Fcn2 : Fcn  Expr=u(1) > pi/6
  Fcn3 : Fcn  Expr=u(1) <= pi/6
  Fcn4 : Fcn  Expr=u(1) >= -pi/6
  Fcn5 : Fcn  Expr="u(1) <=  7*pi/6"
  Fcn6 : Fcn  Expr=u(1) > 5*pi/6
  Fcn7 : Fcn  Expr=u(1) <= 11*pi/6
  Fcn8 : Fcn  Expr=u(1) > 7*pi/6
  Logical Operator{,1..3} (4 alike) : Logic
  Sum1 : Sum  Inputs=++++  InputSameDT=on  SaturateOnIntegerOverflow=on  OutDataTypeStr=Inherit: Same as first input
  Switch{,1..2,5} (4 alike) : Switch  Threshold=.5  SaturateOnIntegerOverflow=on  InputSameDT=on
  interval : Outport
  wires:
  Fcn1/1 -> Logical Operator/2
  Fcn2/1 -> Logical Operator/1
  Logical Operator/1 -> Switch/2
  Fcn5/1 -> Logical Operator1/2
  Fcn6/1 -> Logical Operator1/1
  Logical Operator1/1 -> Switch1/2
  Fcn7/1 -> Logical Operator2/2
  Fcn8/1 -> Logical Operator2/1
  Logical Operator2/1 -> Switch2/2
  Constant4/1 -> Switch1/3
  Constant10/1 -> Switch5/1
  Constant11/1 -> Switch5/3
  Switch1/1 -> Sum1/3
  Switch5/1 -> Sum1/1
  Constant2/1 -> Switch/1
  Constant5/1 -> Switch1/1
  Constant3/1 -> Switch/3
  Constant6/1 -> Switch2/1
  Constant7/1 -> Switch2/3
  Switch/1 -> Sum1/2
  Switch2/1 -> Sum1/4
  -pi/6 < theta < 11pi/6/1 -> Fcn3/1, Fcn2/1, Fcn1/1, Fcn6/1, Fcn5/1, Fcn8/1, Fcn7/1, Fcn4/1
  Sum1/1 -> interval/1
  Logical Operator3/1 -> Switch5/2
  Fcn4/1 -> Logical Operator3/1
  Fcn3/1 -> Logical Operator3/2

== system BldcClosedLoop2/BLDC Motor/Back Emfs/es2/-pi//6 < theta < 11pi//6 ==
  0 < theta < 2pi : Inport
  Constant3 : Constant  Value=2*pi
  Fcn3 : Fcn  Expr="2*pi - u(1) <=  pi/6"
  Sum1 : Sum  Inputs=|-+  InputSameDT=on  SaturateOnIntegerOverflow=on  OutDataTypeStr=Inherit: Same as first input
  Switch1 : Switch  Threshold=.5  SaturateOnIntegerOverflow=on  InputSameDT=on
  -pi/6 < theta < 11pi/6 : Outport
  wires:
  0 < theta < 2pi/1 -> Switch1/3, Fcn3/1, Sum1/2
  Constant3/1 -> Sum1/1
  Switch1/1 -> -pi/6 < theta < 11pi/6/1
  Sum1/1 -> Switch1/1
  Fcn3/1 -> Switch1/2

== system BldcClosedLoop2/BLDC Motor/Back Emfs/es2/0 < theta < 2pi ==
  theta : Inport
  Constant1 : Constant  Value=2*pi
  Fcn4 : Fcn  Expr=rem(u(1),2*pi)
  Scope1 : Scope
  Sum2 : Sum  Inputs=|++  InputSameDT=on  SaturateOnIntegerOverflow=on  OutDataTypeStr=Inherit: Same as first input
  Switch3 : Switch  SaturateOnIntegerOverflow=on  InputSameDT=on
  0 < theta < 2pi : Outport
  wires:
  Sum2/1 -> Switch3/3
  Fcn4/1 -> Sum2/1, Switch3/1, Switch3/2
  Constant1/1 -> Sum2/2
  theta/1 -> Fcn4/1, Scope1/1
  Switch3/1 -> 0 < theta < 2pi/1

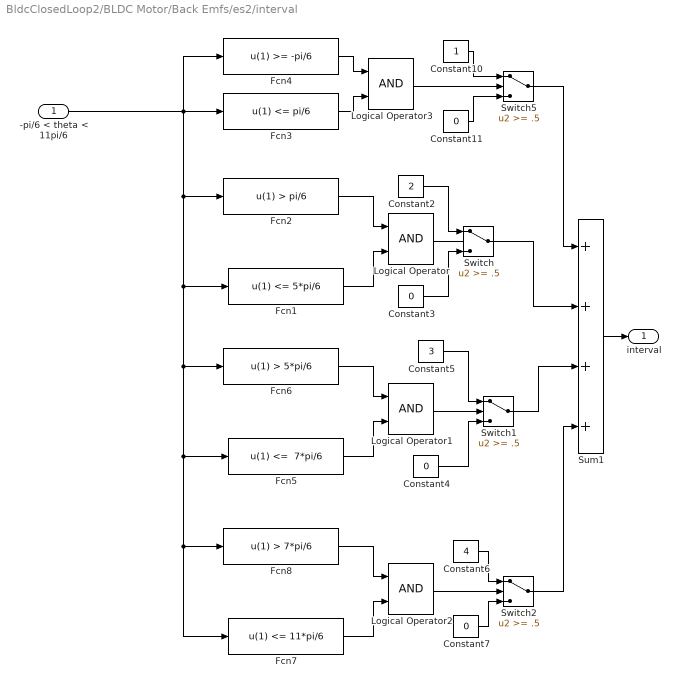
== system BldcClosedLoop2/BLDC Motor/Back Emfs/es2/interval ==
  -pi/6 < theta < 11pi/6 : Inport
  Constant10 : Constant
  Constant{3..4,7,11} (4 alike) : Constant  Value=0
  Constant2 : Constant  Value=2
  Constant5 : Constant  Value=3
  Constant6 : Constant  Value=4
  Fcn1 : Fcn  Expr=u(1) <= 5*pi/6
  Fcn2 : Fcn  Expr=u(1) > pi/6
  Fcn3 : Fcn  Expr=u(1) <= pi/6
  Fcn4 : Fcn  Expr=u(1) >= -pi/6
  Fcn5 : Fcn  Expr="u(1) <=  7*pi/6"
  Fcn6 : Fcn  Expr=u(1) > 5*pi/6
  Fcn7 : Fcn  Expr=u(1) <= 11*pi/6
  Fcn8 : Fcn  Expr=u(1) > 7*pi/6
  Logical Operator{,1..3} (4 alike) : Logic
  Sum1 : Sum  Inputs=++++  InputSameDT=on  SaturateOnIntegerOverflow=on  OutDataTypeStr=Inherit: Same as first input
  Switch{,1..2,5} (4 alike) : Switch  Threshold=.5  SaturateOnIntegerOverflow=on  InputSameDT=on
  interval : Outport
  wires:
  Fcn1/1 -> Logical Operator/2
  Fcn2/1 -> Logical Operator/1
  Logical Operator/1 -> Switch/2
  Fcn5/1 -> Logical Operator1/2
  Fcn6/1 -> Logical Operator1/1
  Logical Operator1/1 -> Switch1/2
  Fcn7/1 -> Logical Operator2/2
  Fcn8/1 -> Logical Operator2/1
  Logical Operator2/1 -> Switch2/2
  Constant4/1 -> Switch1/3
  Constant10/1 -> Switch5/1
  Constant11/1 -> Switch5/3
  Switch1/1 -> Sum1/3
  Switch5/1 -> Sum1/1
  Constant2/1 -> Switch/1
  Constant5/1 -> Switch1/1
  Constant3/1 -> Switch/3
  Constant6/1 -> Switch2/1
  Constant7/1 -> Switch2/3
  Switch/1 -> Sum1/2
  Switch2/1 -> Sum1/4
  -pi/6 < theta < 11pi/6/1 -> Fcn3/1, Fcn2/1, Fcn1/1, Fcn6/1, Fcn5/1, Fcn8/1, Fcn7/1, Fcn4/1
  Sum1/1 -> interval/1
  Logical Operator3/1 -> Switch5/2
  Fcn4/1 -> Logical Operator3/1
  Fcn3/1 -> Logical Operator3/2

== system BldcClosedLoop2/BLDC Motor/Back Emfs/es3/-pi//6 < theta < 11pi//6 ==
  0 < theta < 2pi : Inport
  Constant3 : Constant  Value=2*pi
  Fcn3 : Fcn  Expr="2*pi - u(1) <=  pi/6"
  Sum1 : Sum  Inputs=|-+  InputSameDT=on  SaturateOnIntegerOverflow=on  OutDataTypeStr=Inherit: Same as first input
  Switch1 : Switch  Threshold=.5  SaturateOnIntegerOverflow=on  InputSameDT=on
  -pi/6 < theta < 11pi/6 : Outport
  wires:
  0 < theta < 2pi/1 -> Switch1/3, Fcn3/1, Sum1/2
  Constant3/1 -> Sum1/1
  Switch1/1 -> -pi/6 < theta < 11pi/6/1
  Sum1/1 -> Switch1/1
  Fcn3/1 -> Switch1/2

== system BldcClosedLoop2/BLDC Motor/Back Emfs/es3/0 < theta < 2pi ==
  theta : Inport
  Constant1 : Constant  Value=2*pi
  Fcn4 : Fcn  Expr=rem(u(1),2*pi)
  Scope1 : Scope
  Sum2 : Sum  Inputs=|++  InputSameDT=on  SaturateOnIntegerOverflow=on  OutDataTypeStr=Inherit: Same as first input
  Switch3 : Switch  SaturateOnIntegerOverflow=on  InputSameDT=on
  0 < theta < 2pi : Outport
  wires:
  Sum2/1 -> Switch3/3
  Fcn4/1 -> Sum2/1, Switch3/1, Switch3/2
  Constant1/1 -> Sum2/2
  theta/1 -> Fcn4/1, Scope1/1
  Switch3/1 -> 0 < theta < 2pi/1

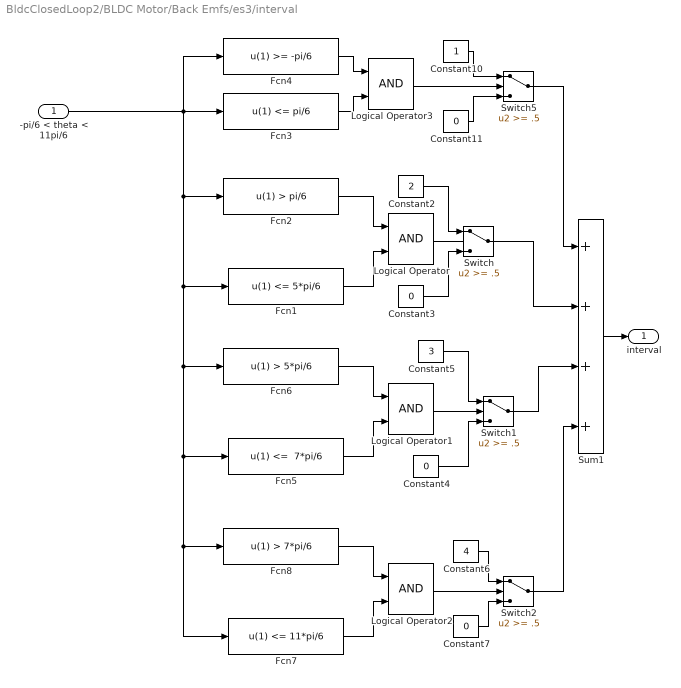
== system BldcClosedLoop2/BLDC Motor/Back Emfs/es3/interval ==
  -pi/6 < theta < 11pi/6 : Inport
  Constant10 : Constant
  Constant{3..4,7,11} (4 alike) : Constant  Value=0
  Constant2 : Constant  Value=2
  Constant5 : Constant  Value=3
  Constant6 : Constant  Value=4
  Fcn1 : Fcn  Expr=u(1) <= 5*pi/6
  Fcn2 : Fcn  Expr=u(1) > pi/6
  Fcn3 : Fcn  Expr=u(1) <= pi/6
  Fcn4 : Fcn  Expr=u(1) >= -pi/6
  Fcn5 : Fcn  Expr="u(1) <=  7*pi/6"
  Fcn6 : Fcn  Expr=u(1) > 5*pi/6
  Fcn7 : Fcn  Expr=u(1) <= 11*pi/6
  Fcn8 : Fcn  Expr=u(1) > 7*pi/6
  Logical Operator{,1..3} (4 alike) : Logic
  Sum1 : Sum  Inputs=++++  InputSameDT=on  SaturateOnIntegerOverflow=on  OutDataTypeStr=Inherit: Same as first input
  Switch{,1..2,5} (4 alike) : Switch  Threshold=.5  SaturateOnIntegerOverflow=on  InputSameDT=on
  interval : Outport
  wires:
  Fcn1/1 -> Logical Operator/2
  Fcn2/1 -> Logical Operator/1
  Logical Operator/1 -> Switch/2
  Fcn5/1 -> Logical Operator1/2
  Fcn6/1 -> Logical Operator1/1
  Logical Operator1/1 -> Switch1/2
  Fcn7/1 -> Logical Operator2/2
  Fcn8/1 -> Logical Operator2/1
  Logical Operator2/1 -> Switch2/2
  Constant4/1 -> Switch1/3
  Constant10/1 -> Switch5/1
  Constant11/1 -> Switch5/3
  Switch1/1 -> Sum1/3
  Switch5/1 -> Sum1/1
  Constant2/1 -> Switch/1
  Constant5/1 -> Switch1/1
  Constant3/1 -> Switch/3
  Constant6/1 -> Switch2/1
  Constant7/1 -> Switch2/3
  Switch/1 -> Sum1/2
  Switch2/1 -> Sum1/4
  -pi/6 < theta < 11pi/6/1 -> Fcn3/1, Fcn2/1, Fcn1/1, Fcn6/1, Fcn5/1, Fcn8/1, Fcn7/1, Fcn4/1
  Sum1/1 -> interval/1
  Logical Operator3/1 -> Switch5/2
  Fcn4/1 -> Logical Operator3/1
  Fcn3/1 -> Logical Operator3/2

== system BldcClosedLoop2/BLDC Motor/Phase Torques/Tau1/-pi//6 < theta < 11pi//6  ==
  0 < theta < 2pi : Inport
  Constant3 : Constant  Value=2*pi
  Fcn3 : Fcn  Expr="2*pi - u(1) <=  pi/6"
  Sum1 : Sum  Inputs=|-+  InputSameDT=on  SaturateOnIntegerOverflow=on  OutDataTypeStr=Inherit: Same as first input
  Switch1 : Switch  Threshold=.5  SaturateOnIntegerOverflow=on  InputSameDT=on
  -pi/6 < theta < 11pi/6 : Outport
  wires:
  0 < theta < 2pi/1 -> Switch1/3, Fcn3/1, Sum1/2
  Constant3/1 -> Sum1/1
  Switch1/1 -> -pi/6 < theta < 11pi/6/1
  Sum1/1 -> Switch1/1
  Fcn3/1 -> Switch1/2

== system BldcClosedLoop2/BLDC Motor/Phase Torques/Tau1/0 < theta < 2pi ==
  theta : Inport
  Constant1 : Constant  Value=2*pi
  Fcn4 : Fcn  Expr=rem(u(1),2*pi)
  Scope1 : Scope
  Sum2 : Sum  Inputs=|++  InputSameDT=on  SaturateOnIntegerOverflow=on  OutDataTypeStr=Inherit: Same as first input
  Switch3 : Switch  SaturateOnIntegerOverflow=on  InputSameDT=on
  0 < theta < 2pi : Outport
  wires:
  Sum2/1 -> Switch3/3
  Fcn4/1 -> Sum2/1, Switch3/1, Switch3/2
  Constant1/1 -> Sum2/2
  theta/1 -> Fcn4/1, Scope1/1
  Switch3/1 -> 0 < theta < 2pi/1

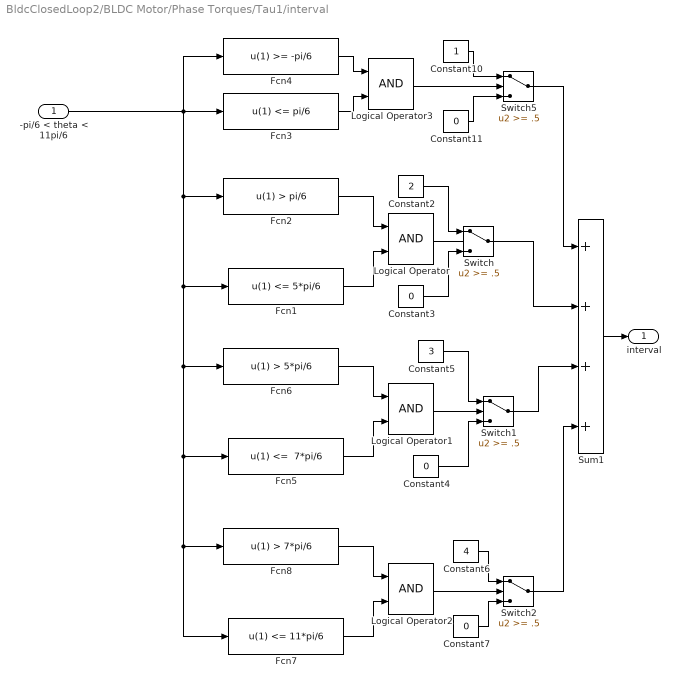
== system BldcClosedLoop2/BLDC Motor/Phase Torques/Tau1/interval ==
  -pi/6 < theta < 11pi/6 : Inport
  Constant10 : Constant
  Constant{3..4,7,11} (4 alike) : Constant  Value=0
  Constant2 : Constant  Value=2
  Constant5 : Constant  Value=3
  Constant6 : Constant  Value=4
  Fcn1 : Fcn  Expr=u(1) <= 5*pi/6
  Fcn2 : Fcn  Expr=u(1) > pi/6
  Fcn3 : Fcn  Expr=u(1) <= pi/6
  Fcn4 : Fcn  Expr=u(1) >= -pi/6
  Fcn5 : Fcn  Expr="u(1) <=  7*pi/6"
  Fcn6 : Fcn  Expr=u(1) > 5*pi/6
  Fcn7 : Fcn  Expr=u(1) <= 11*pi/6
  Fcn8 : Fcn  Expr=u(1) > 7*pi/6
  Logical Operator{,1..3} (4 alike) : Logic
  Sum1 : Sum  Inputs=++++  InputSameDT=on  SaturateOnIntegerOverflow=on  OutDataTypeStr=Inherit: Same as first input
  Switch{,1..2,5} (4 alike) : Switch  Threshold=.5  SaturateOnIntegerOverflow=on  InputSameDT=on
  interval : Outport
  wires:
  Fcn1/1 -> Logical Operator/2
  Fcn2/1 -> Logical Operator/1
  Logical Operator/1 -> Switch/2
  Fcn5/1 -> Logical Operator1/2
  Fcn6/1 -> Logical Operator1/1
  Logical Operator1/1 -> Switch1/2
  Fcn7/1 -> Logical Operator2/2
  Fcn8/1 -> Logical Operator2/1
  Logical Operator2/1 -> Switch2/2
  Constant4/1 -> Switch1/3
  Constant10/1 -> Switch5/1
  Constant11/1 -> Switch5/3
  Switch1/1 -> Sum1/3
  Switch5/1 -> Sum1/1
  Constant2/1 -> Switch/1
  Constant5/1 -> Switch1/1
  Constant3/1 -> Switch/3
  Constant6/1 -> Switch2/1
  Constant7/1 -> Switch2/3
  Switch/1 -> Sum1/2
  Switch2/1 -> Sum1/4
  -pi/6 < theta < 11pi/6/1 -> Fcn3/1, Fcn2/1, Fcn1/1, Fcn6/1, Fcn5/1, Fcn8/1, Fcn7/1, Fcn4/1
  Sum1/1 -> interval/1
  Logical Operator3/1 -> Switch5/2
  Fcn4/1 -> Logical Operator3/1
  Fcn3/1 -> Logical Operator3/2

== system BldcClosedLoop2/BLDC Motor/Phase Torques/Tau2/-pi//6 < theta < 11pi//6 ==
  0 < theta < 2pi : Inport
  Constant3 : Constant  Value=2*pi
  Fcn3 : Fcn  Expr="2*pi - u(1) <=  pi/6"
  Sum1 : Sum  Inputs=|-+  InputSameDT=on  SaturateOnIntegerOverflow=on  OutDataTypeStr=Inherit: Same as first input
  Switch1 : Switch  Threshold=.5  SaturateOnIntegerOverflow=on  InputSameDT=on
  -pi/6 < theta < 11pi/6 : Outport
  wires:
  0 < theta < 2pi/1 -> Switch1/3, Fcn3/1, Sum1/2
  Constant3/1 -> Sum1/1
  Switch1/1 -> -pi/6 < theta < 11pi/6/1
  Sum1/1 -> Switch1/1
  Fcn3/1 -> Switch1/2

== system BldcClosedLoop2/BLDC Motor/Phase Torques/Tau2/0 < theta < 2pi ==
  theta : Inport
  Constant1 : Constant  Value=2*pi
  Fcn4 : Fcn  Expr=rem(u(1),2*pi)
  Scope1 : Scope
  Sum2 : Sum  Inputs=|++  InputSameDT=on  SaturateOnIntegerOverflow=on  OutDataTypeStr=Inherit: Same as first input
  Switch3 : Switch  SaturateOnIntegerOverflow=on  InputSameDT=on
  0 < theta < 2pi : Outport
  wires:
  Sum2/1 -> Switch3/3
  Fcn4/1 -> Sum2/1, Switch3/1, Switch3/2
  Constant1/1 -> Sum2/2
  theta/1 -> Fcn4/1, Scope1/1
  Switch3/1 -> 0 < theta < 2pi/1

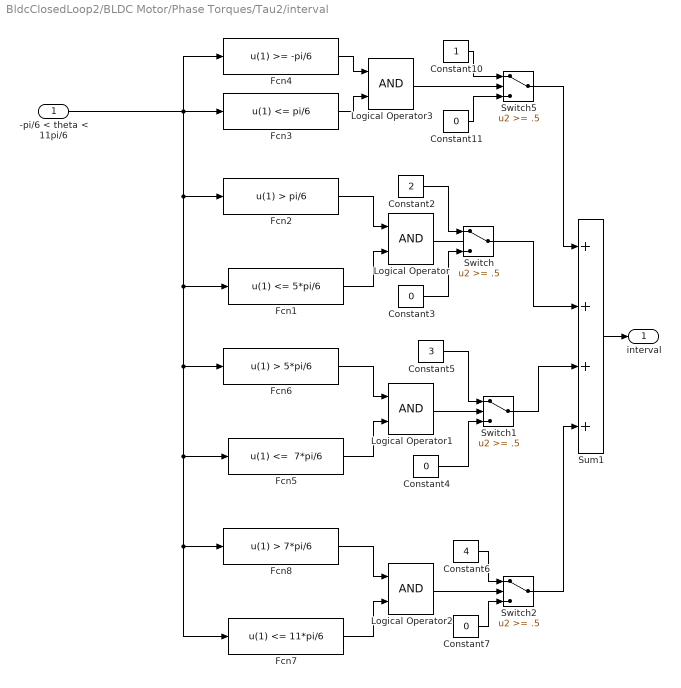
== system BldcClosedLoop2/BLDC Motor/Phase Torques/Tau2/interval ==
  -pi/6 < theta < 11pi/6 : Inport
  Constant10 : Constant
  Constant{3..4,7,11} (4 alike) : Constant  Value=0
  Constant2 : Constant  Value=2
  Constant5 : Constant  Value=3
  Constant6 : Constant  Value=4
  Fcn1 : Fcn  Expr=u(1) <= 5*pi/6
  Fcn2 : Fcn  Expr=u(1) > pi/6
  Fcn3 : Fcn  Expr=u(1) <= pi/6
  Fcn4 : Fcn  Expr=u(1) >= -pi/6
  Fcn5 : Fcn  Expr="u(1) <=  7*pi/6"
  Fcn6 : Fcn  Expr=u(1) > 5*pi/6
  Fcn7 : Fcn  Expr=u(1) <= 11*pi/6
  Fcn8 : Fcn  Expr=u(1) > 7*pi/6
  Logical Operator{,1..3} (4 alike) : Logic
  Sum1 : Sum  Inputs=++++  InputSameDT=on  SaturateOnIntegerOverflow=on  OutDataTypeStr=Inherit: Same as first input
  Switch{,1..2,5} (4 alike) : Switch  Threshold=.5  SaturateOnIntegerOverflow=on  InputSameDT=on
  interval : Outport
  wires:
  Fcn1/1 -> Logical Operator/2
  Fcn2/1 -> Logical Operator/1
  Logical Operator/1 -> Switch/2
  Fcn5/1 -> Logical Operator1/2
  Fcn6/1 -> Logical Operator1/1
  Logical Operator1/1 -> Switch1/2
  Fcn7/1 -> Logical Operator2/2
  Fcn8/1 -> Logical Operator2/1
  Logical Operator2/1 -> Switch2/2
  Constant4/1 -> Switch1/3
  Constant10/1 -> Switch5/1
  Constant11/1 -> Switch5/3
  Switch1/1 -> Sum1/3
  Switch5/1 -> Sum1/1
  Constant2/1 -> Switch/1
  Constant5/1 -> Switch1/1
  Constant3/1 -> Switch/3
  Constant6/1 -> Switch2/1
  Constant7/1 -> Switch2/3
  Switch/1 -> Sum1/2
  Switch2/1 -> Sum1/4
  -pi/6 < theta < 11pi/6/1 -> Fcn3/1, Fcn2/1, Fcn1/1, Fcn6/1, Fcn5/1, Fcn8/1, Fcn7/1, Fcn4/1
  Sum1/1 -> interval/1
  Logical Operator3/1 -> Switch5/2
  Fcn4/1 -> Logical Operator3/1
  Fcn3/1 -> Logical Operator3/2

== system BldcClosedLoop2/BLDC Motor/Phase Torques/Tau3/-pi//6 < theta < 11pi//6 ==
  0 < theta < 2pi : Inport
  Constant3 : Constant  Value=2*pi
  Fcn3 : Fcn  Expr="2*pi - u(1) <=  pi/6"
  Sum1 : Sum  Inputs=|-+  InputSameDT=on  SaturateOnIntegerOverflow=on  OutDataTypeStr=Inherit: Same as first input
  Switch1 : Switch  Threshold=.5  SaturateOnIntegerOverflow=on  InputSameDT=on
  -pi/6 < theta < 11pi/6 : Outport
  wires:
  0 < theta < 2pi/1 -> Switch1/3, Fcn3/1, Sum1/2
  Constant3/1 -> Sum1/1
  Switch1/1 -> -pi/6 < theta < 11pi/6/1
  Sum1/1 -> Switch1/1
  Fcn3/1 -> Switch1/2

== system BldcClosedLoop2/BLDC Motor/Phase Torques/Tau3/0 < theta < 2pi ==
  theta : Inport
  Constant1 : Constant  Value=2*pi
  Fcn4 : Fcn  Expr=rem(u(1),2*pi)
  Scope1 : Scope
  Sum2 : Sum  Inputs=|++  InputSameDT=on  SaturateOnIntegerOverflow=on  OutDataTypeStr=Inherit: Same as first input
  Switch3 : Switch  SaturateOnIntegerOverflow=on  InputSameDT=on
  0 < theta < 2pi : Outport
  wires:
  Sum2/1 -> Switch3/3
  Fcn4/1 -> Sum2/1, Switch3/1, Switch3/2
  Constant1/1 -> Sum2/2
  theta/1 -> Fcn4/1, Scope1/1
  Switch3/1 -> 0 < theta < 2pi/1

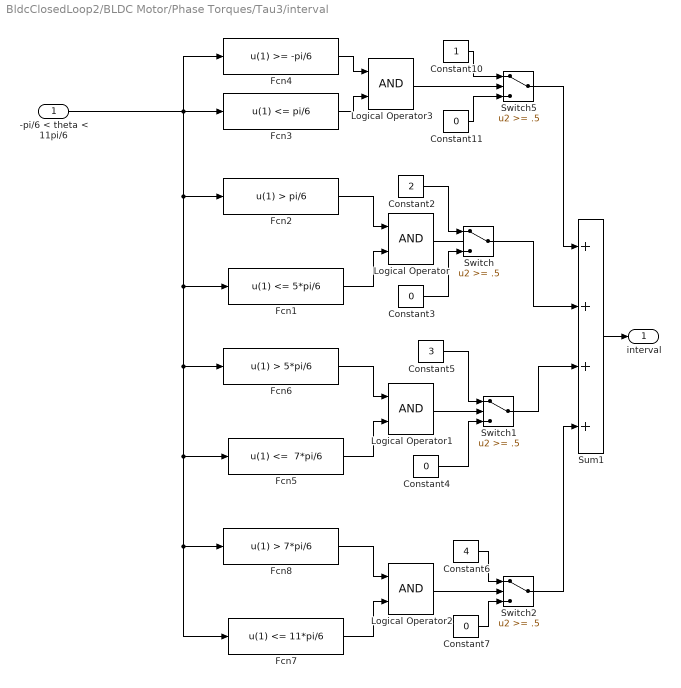
== system BldcClosedLoop2/BLDC Motor/Phase Torques/Tau3/interval ==
  -pi/6 < theta < 11pi/6 : Inport
  Constant10 : Constant
  Constant{3..4,7,11} (4 alike) : Constant  Value=0
  Constant2 : Constant  Value=2
  Constant5 : Constant  Value=3
  Constant6 : Constant  Value=4
  Fcn1 : Fcn  Expr=u(1) <= 5*pi/6
  Fcn2 : Fcn  Expr=u(1) > pi/6
  Fcn3 : Fcn  Expr=u(1) <= pi/6
  Fcn4 : Fcn  Expr=u(1) >= -pi/6
  Fcn5 : Fcn  Expr="u(1) <=  7*pi/6"
  Fcn6 : Fcn  Expr=u(1) > 5*pi/6
  Fcn7 : Fcn  Expr=u(1) <= 11*pi/6
  Fcn8 : Fcn  Expr=u(1) > 7*pi/6
  Logical Operator{,1..3} (4 alike) : Logic
  Sum1 : Sum  Inputs=++++  InputSameDT=on  SaturateOnIntegerOverflow=on  OutDataTypeStr=Inherit: Same as first input
  Switch{,1..2,5} (4 alike) : Switch  Threshold=.5  SaturateOnIntegerOverflow=on  InputSameDT=on
  interval : Outport
  wires:
  Fcn1/1 -> Logical Operator/2
  Fcn2/1 -> Logical Operator/1
  Logical Operator/1 -> Switch/2
  Fcn5/1 -> Logical Operator1/2
  Fcn6/1 -> Logical Operator1/1
  Logical Operator1/1 -> Switch1/2
  Fcn7/1 -> Logical Operator2/2
  Fcn8/1 -> Logical Operator2/1
  Logical Operator2/1 -> Switch2/2
  Constant4/1 -> Switch1/3
  Constant10/1 -> Switch5/1
  Constant11/1 -> Switch5/3
  Switch1/1 -> Sum1/3
  Switch5/1 -> Sum1/1
  Constant2/1 -> Switch/1
  Constant5/1 -> Switch1/1
  Constant3/1 -> Switch/3
  Constant6/1 -> Switch2/1
  Constant7/1 -> Switch2/3
  Switch/1 -> Sum1/2
  Switch2/1 -> Sum1/4
  -pi/6 < theta < 11pi/6/1 -> Fcn3/1, Fcn2/1, Fcn1/1, Fcn6/1, Fcn5/1, Fcn8/1, Fcn7/1, Fcn4/1
  Sum1/1 -> interval/1
  Logical Operator3/1 -> Switch5/2
  Fcn4/1 -> Logical Operator3/1
  Fcn3/1 -> Logical Operator3/2

== system BldcClosedLoop2/Controller/current commands/IS1c/-pi//6 < theta < 11pi//6  ==
  0 < theta < 2pi : Inport
  Constant3 : Constant  Value=2*pi
  Fcn3 : Fcn  Expr="2*pi - u(1) <=  pi/6"
  Sum1 : Sum  Inputs=|-+  InputSameDT=on  SaturateOnIntegerOverflow=on  OutDataTypeStr=Inherit: Same as first input
  Switch1 : Switch  Threshold=.5  SaturateOnIntegerOverflow=on  InputSameDT=on
  -pi/6 < theta < 11pi/6 : Outport
  wires:
  0 < theta < 2pi/1 -> Switch1/3, Fcn3/1, Sum1/2
  Constant3/1 -> Sum1/1
  Switch1/1 -> -pi/6 < theta < 11pi/6/1
  Sum1/1 -> Switch1/1
  Fcn3/1 -> Switch1/2

== system BldcClosedLoop2/Controller/current commands/IS1c/0 < theta < 2pi ==
  theta : Inport
  Constant1 : Constant  Value=2*pi
  Fcn4 : Fcn  Expr=rem(u(1),2*pi)
  Scope1 : Scope
  Sum2 : Sum  Inputs=|++  InputSameDT=on  SaturateOnIntegerOverflow=on  OutDataTypeStr=Inherit: Same as first input
  Switch3 : Switch  SaturateOnIntegerOverflow=on  InputSameDT=on
  0 < theta < 2pi : Outport
  wires:
  Sum2/1 -> Switch3/3
  Fcn4/1 -> Sum2/1, Switch3/1, Switch3/2
  Constant1/1 -> Sum2/2
  theta/1 -> Fcn4/1, Scope1/1
  Switch3/1 -> 0 < theta < 2pi/1

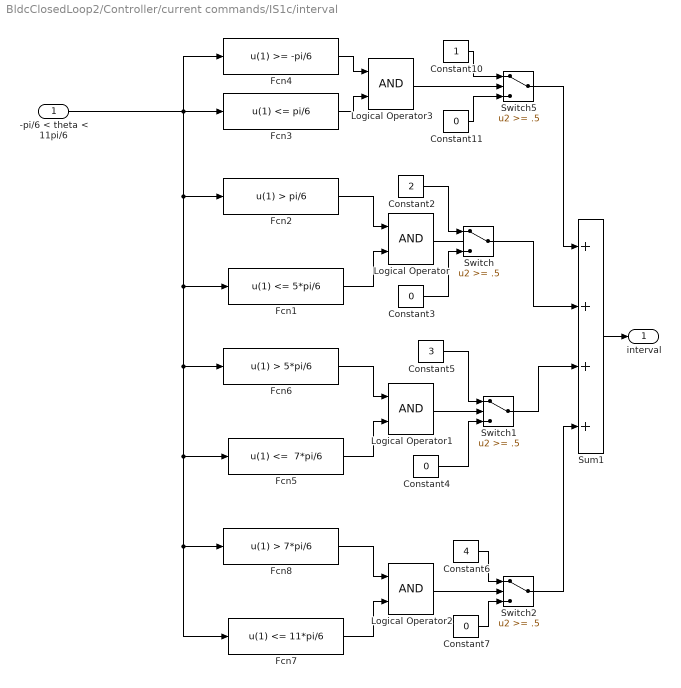
== system BldcClosedLoop2/Controller/current commands/IS1c/interval ==
  -pi/6 < theta < 11pi/6 : Inport
  Constant10 : Constant
  Constant{3..4,7,11} (4 alike) : Constant  Value=0
  Constant2 : Constant  Value=2
  Constant5 : Constant  Value=3
  Constant6 : Constant  Value=4
  Fcn1 : Fcn  Expr=u(1) <= 5*pi/6
  Fcn2 : Fcn  Expr=u(1) > pi/6
  Fcn3 : Fcn  Expr=u(1) <= pi/6
  Fcn4 : Fcn  Expr=u(1) >= -pi/6
  Fcn5 : Fcn  Expr="u(1) <=  7*pi/6"
  Fcn6 : Fcn  Expr=u(1) > 5*pi/6
  Fcn7 : Fcn  Expr=u(1) <= 11*pi/6
  Fcn8 : Fcn  Expr=u(1) > 7*pi/6
  Logical Operator{,1..3} (4 alike) : Logic
  Sum1 : Sum  Inputs=++++  InputSameDT=on  SaturateOnIntegerOverflow=on  OutDataTypeStr=Inherit: Same as first input
  Switch{,1..2,5} (4 alike) : Switch  Threshold=.5  SaturateOnIntegerOverflow=on  InputSameDT=on
  interval : Outport
  wires:
  Fcn1/1 -> Logical Operator/2
  Fcn2/1 -> Logical Operator/1
  Logical Operator/1 -> Switch/2
  Fcn5/1 -> Logical Operator1/2
  Fcn6/1 -> Logical Operator1/1
  Logical Operator1/1 -> Switch1/2
  Fcn7/1 -> Logical Operator2/2
  Fcn8/1 -> Logical Operator2/1
  Logical Operator2/1 -> Switch2/2
  Constant4/1 -> Switch1/3
  Constant10/1 -> Switch5/1
  Constant11/1 -> Switch5/3
  Switch1/1 -> Sum1/3
  Switch5/1 -> Sum1/1
  Constant2/1 -> Switch/1
  Constant5/1 -> Switch1/1
  Constant3/1 -> Switch/3
  Constant6/1 -> Switch2/1
  Constant7/1 -> Switch2/3
  Switch/1 -> Sum1/2
  Switch2/1 -> Sum1/4
  -pi/6 < theta < 11pi/6/1 -> Fcn3/1, Fcn2/1, Fcn1/1, Fcn6/1, Fcn5/1, Fcn8/1, Fcn7/1, Fcn4/1
  Sum1/1 -> interval/1
  Logical Operator3/1 -> Switch5/2
  Fcn4/1 -> Logical Operator3/1
  Fcn3/1 -> Logical Operator3/2

== system BldcClosedLoop2/Controller/current commands/IS2c/-pi//6 < theta < 11pi//6 ==
  0 < theta < 2pi : Inport
  Constant3 : Constant  Value=2*pi
  Fcn3 : Fcn  Expr="2*pi - u(1) <=  pi/6"
  Sum1 : Sum  Inputs=|-+  InputSameDT=on  SaturateOnIntegerOverflow=on  OutDataTypeStr=Inherit: Same as first input
  Switch1 : Switch  Threshold=.5  SaturateOnIntegerOverflow=on  InputSameDT=on
  -pi/6 < theta < 11pi/6 : Outport
  wires:
  0 < theta < 2pi/1 -> Switch1/3, Fcn3/1, Sum1/2
  Constant3/1 -> Sum1/1
  Switch1/1 -> -pi/6 < theta < 11pi/6/1
  Sum1/1 -> Switch1/1
  Fcn3/1 -> Switch1/2

== system BldcClosedLoop2/Controller/current commands/IS2c/0 < theta < 2pi ==
  theta : Inport
  Constant1 : Constant  Value=2*pi
  Fcn4 : Fcn  Expr=rem(u(1),2*pi)
  Scope1 : Scope
  Sum2 : Sum  Inputs=|++  InputSameDT=on  SaturateOnIntegerOverflow=on  OutDataTypeStr=Inherit: Same as first input
  Switch3 : Switch  SaturateOnIntegerOverflow=on  InputSameDT=on
  0 < theta < 2pi : Outport
  wires:
  Sum2/1 -> Switch3/3
  Fcn4/1 -> Sum2/1, Switch3/1, Switch3/2
  Constant1/1 -> Sum2/2
  theta/1 -> Fcn4/1, Scope1/1
  Switch3/1 -> 0 < theta < 2pi/1

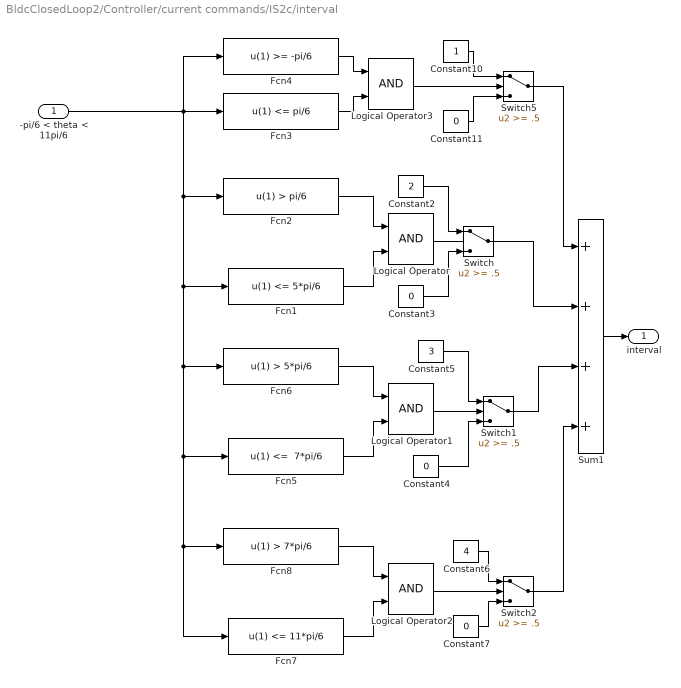
== system BldcClosedLoop2/Controller/current commands/IS2c/interval ==
  -pi/6 < theta < 11pi/6 : Inport
  Constant10 : Constant
  Constant{3..4,7,11} (4 alike) : Constant  Value=0
  Constant2 : Constant  Value=2
  Constant5 : Constant  Value=3
  Constant6 : Constant  Value=4
  Fcn1 : Fcn  Expr=u(1) <= 5*pi/6
  Fcn2 : Fcn  Expr=u(1) > pi/6
  Fcn3 : Fcn  Expr=u(1) <= pi/6
  Fcn4 : Fcn  Expr=u(1) >= -pi/6
  Fcn5 : Fcn  Expr="u(1) <=  7*pi/6"
  Fcn6 : Fcn  Expr=u(1) > 5*pi/6
  Fcn7 : Fcn  Expr=u(1) <= 11*pi/6
  Fcn8 : Fcn  Expr=u(1) > 7*pi/6
  Logical Operator{,1..3} (4 alike) : Logic
  Sum1 : Sum  Inputs=++++  InputSameDT=on  SaturateOnIntegerOverflow=on  OutDataTypeStr=Inherit: Same as first input
  Switch{,1..2,5} (4 alike) : Switch  Threshold=.5  SaturateOnIntegerOverflow=on  InputSameDT=on
  interval : Outport
  wires:
  Fcn1/1 -> Logical Operator/2
  Fcn2/1 -> Logical Operator/1
  Logical Operator/1 -> Switch/2
  Fcn5/1 -> Logical Operator1/2
  Fcn6/1 -> Logical Operator1/1
  Logical Operator1/1 -> Switch1/2
  Fcn7/1 -> Logical Operator2/2
  Fcn8/1 -> Logical Operator2/1
  Logical Operator2/1 -> Switch2/2
  Constant4/1 -> Switch1/3
  Constant10/1 -> Switch5/1
  Constant11/1 -> Switch5/3
  Switch1/1 -> Sum1/3
  Switch5/1 -> Sum1/1
  Constant2/1 -> Switch/1
  Constant5/1 -> Switch1/1
  Constant3/1 -> Switch/3
  Constant6/1 -> Switch2/1
  Constant7/1 -> Switch2/3
  Switch/1 -> Sum1/2
  Switch2/1 -> Sum1/4
  -pi/6 < theta < 11pi/6/1 -> Fcn3/1, Fcn2/1, Fcn1/1, Fcn6/1, Fcn5/1, Fcn8/1, Fcn7/1, Fcn4/1
  Sum1/1 -> interval/1
  Logical Operator3/1 -> Switch5/2
  Fcn4/1 -> Logical Operator3/1
  Fcn3/1 -> Logical Operator3/2

== system BldcClosedLoop2/Controller/current commands/IS3c/-pi//6 < theta < 11pi//6 ==
  0 < theta < 2pi : Inport
  Constant3 : Constant  Value=2*pi
  Fcn3 : Fcn  Expr="2*pi - u(1) <=  pi/6"
  Sum1 : Sum  Inputs=|-+  InputSameDT=on  SaturateOnIntegerOverflow=on  OutDataTypeStr=Inherit: Same as first input
  Switch1 : Switch  Threshold=.5  SaturateOnIntegerOverflow=on  InputSameDT=on
  -pi/6 < theta < 11pi/6 : Outport
  wires:
  0 < theta < 2pi/1 -> Switch1/3, Fcn3/1, Sum1/2
  Constant3/1 -> Sum1/1
  Switch1/1 -> -pi/6 < theta < 11pi/6/1
  Sum1/1 -> Switch1/1
  Fcn3/1 -> Switch1/2
